simulink model "PCM Circuit"  (R2022b)
settings: Solver=VariableStepAuto  StartTime=0.0  StopTime=0.05  RelTol=1e-3
libraries: simulink x2, dspquant2 x2, dspsigops x1
settings Model: Creator=legion  LastModifiedBy=legion

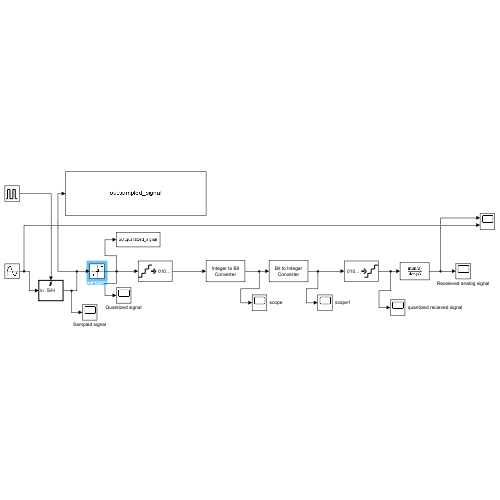
[thumbnail: Simulink's stored preview of the top-level diagram]
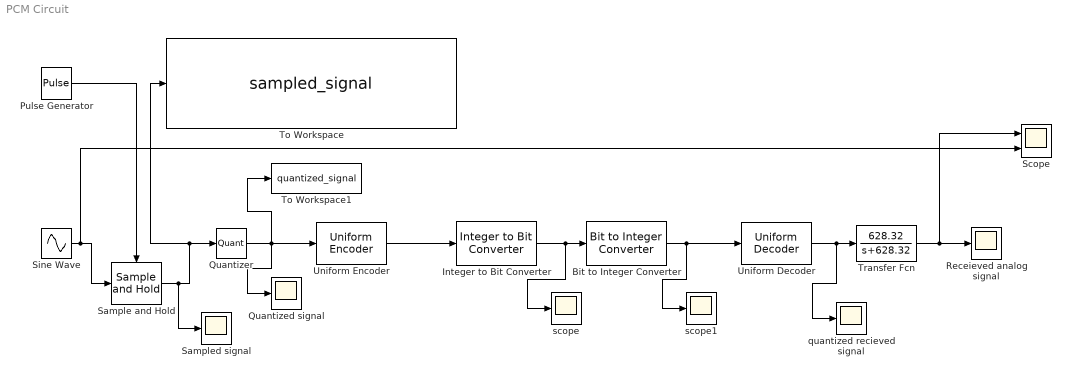
== system PCM Circuit ==
  Bit to Integer Converter : simulink/Logic and Bit Operations/Bit to Integer Converter  nbits=8  bitOrder=MSB first  signedOutputValues=Unsigned  outDtype=Inherit via internal rule  outDtypeSigned=Inherit via internal rule
  Integer to Bit Converter : simulink/Logic and Bit Operations/Integer to Bit Converter  nbits=8  signedInputValues=Unsigned  bitOrder=MSB first  outDtype=Inherit via internal rule
  Pulse Generator : DiscretePulseGenerator  PulseType=Time based  Period=1/8000
  Quantized signal : Scope
  Quantizer : Quantizer  QuantizationInterval=0.0078125  LinearizeAsGain=off
  Receieved analog signal : Scope
  Sample and Hold : dspsigops/Sample and Hold  trig=Rising edge  initCond=0  latchinput=off
  Sampled signal : Scope
  Scope : Scope  NumInputPorts=2
  Sine Wave : Sin  Frequency=628.32  SampleTime=0
  To Workspace : ToWorkspace  VariableName=sampled_signal  SampleTime=-1
  To Workspace1 : ToWorkspace  VariableName=quantized_signal  SampleTime=-1
  Transfer Fcn : TransferFcn  Numerator=[628.32]  Denominator=[1 628.32]
  Uniform Decoder : dspquant2/Uniform Decoder  peak=1  bits=8  overflowMode=Saturate  otype=Double
  Uniform Encoder : dspquant2/Uniform Encoder  peak=1  bits=8  otype=Unsigned integer
  quantized recieved signal : Scope
  scope : Scope
  scope1 : Scope
  wires:
  Sample and Hold/1 -> Sampled signal/1, To Workspace/1, Quantizer/1
  Transfer Fcn/1 -> Scope/1, Receieved analog signal/1
  Sine Wave/1 -> Scope/2, Sample and Hold/1
  Pulse Generator/1 -> Sample and Hold/Trigger
  Quantizer/1 -> To Workspace1/1, Quantized signal/1, Uniform Encoder/1
  Uniform Encoder/1 -> Integer to Bit Converter/1
  Integer to Bit Converter/1 -> scope/1, Bit to Integer Converter/1
  Bit to Integer Converter/1 -> scope1/1, Uniform Decoder/1
  Uniform Decoder/1 -> quantized recieved signal/1, Transfer Fcn/1
